simulink model "chap4_12sim"  (Simulink 5.0)
settings: Solver=ode45  StartTime=0.0  StopTime=5  FixedStep=0.1  RelTol=1e-3
settings Model: LastModifiedBy=Administrator  ExtModeTrigMode=oneshot  ExtModeArmWhenConnect=off  LimitDataPoints=off  BooleanDataType=off

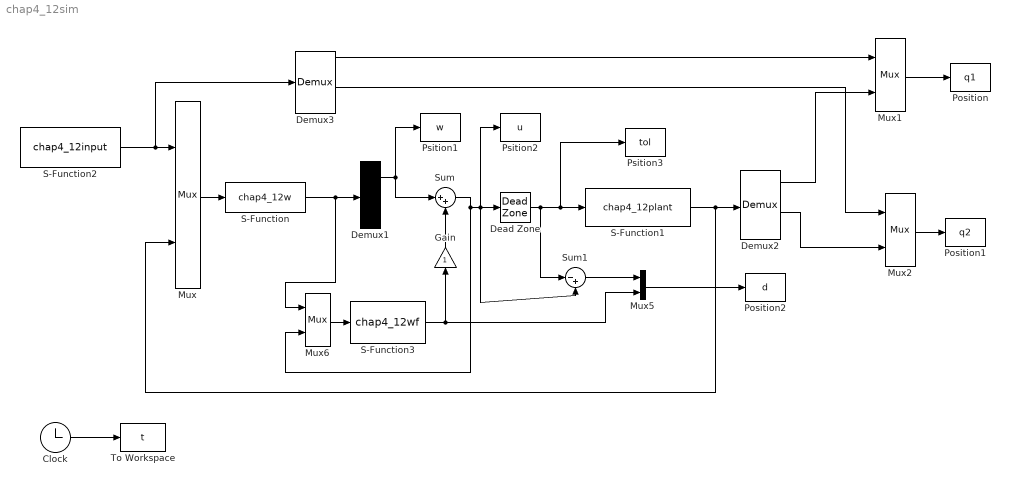
== system chap4_12sim ==
  Clock : Clock
      settings: Decimation=10
  Dead Zone : DeadZone  LowerValue=-15  UpperValue=15  SaturateOnIntegerOverflow=on
  Demux1 : Demux  Outputs=2
  Demux2 : Demux
  Demux3 : Demux  Outputs=6
  Gain : Gain  Orientation=up  SaturateOnIntegerOverflow=on
  Mux{,1..2,5..6} (5 alike) : Mux  Inputs=2
  Position : ToWorkspace  VariableName=q1  SampleTime=-1  SaveFormat=Array
  Position1 : ToWorkspace  VariableName=q2  SampleTime=-1  SaveFormat=Array
  Position2 : ToWorkspace  VariableName=d  SampleTime=-1  SaveFormat=Array
  Psition1 : ToWorkspace  VariableName=w  SampleTime=-1  SaveFormat=Array
  Psition2 : ToWorkspace  VariableName=u  SampleTime=-1  SaveFormat=Array
  Psition3 : ToWorkspace  VariableName=tol  SampleTime=-1  SaveFormat=Array
  S-Function : S-Function  FunctionName=chap4_12w
  S-Function1 : S-Function  FunctionName=chap4_12plant
  S-Function2 : S-Function  FunctionName=chap4_12input
  S-Function3 : S-Function  FunctionName=chap4_12wf
  Sum : Sum  Inputs=|++  SaturateOnIntegerOverflow=on
  Sum1 : Sum  Inputs=|-+  SaturateOnIntegerOverflow=on
  To Workspace : ToWorkspace  VariableName=t  SampleTime=-1  SaveFormat=Array
  wires:
  S-Function/1 -> Mux6/1, Demux1/1
  Demux2/1 -> Mux1/2
  S-Function2/1 -> Demux3/1, Mux/1
  Demux3/1 -> Mux1/1
  S-Function1/1 -> Mux/2, Demux2/1
  Dead Zone/1 -> S-Function1/1, Psition3/1, Sum1/1
  Sum/1 -> Dead Zone/1, Sum1/2, Psition2/1, Mux6/2
  S-Function3/1 -> Gain/1, Mux5/2
  Mux6/1 -> S-Function3/1
  Mux1/1 -> Position/1
  Mux/1 -> S-Function/1
  Mux5/1 -> Position2/1
  Sum1/1 -> Mux5/1
  Clock/1 -> To Workspace/1
  Demux1/1 -> Psition1/1, Sum/1
  Gain/1 -> Sum/2
  Mux2/1 -> Position1/1
  Demux3/4 -> Mux2/1
  Demux2/3 -> Mux2/2
